simulink model "gm_parallel_8_prediction_and_cost_function"  (R2022a)
settings: Solver=FixedStepDiscrete  StartTime=0.0  StopTime=10.0  RelTol=1e-3
undefined symbols (not defined in the file or in its folder): f_c, L_d, L_q, L_x, L_y, p, psi_pm, R_ph
libraries: hdlmdlgenlib x42, hdlsllib x5
(part 2 of 7)

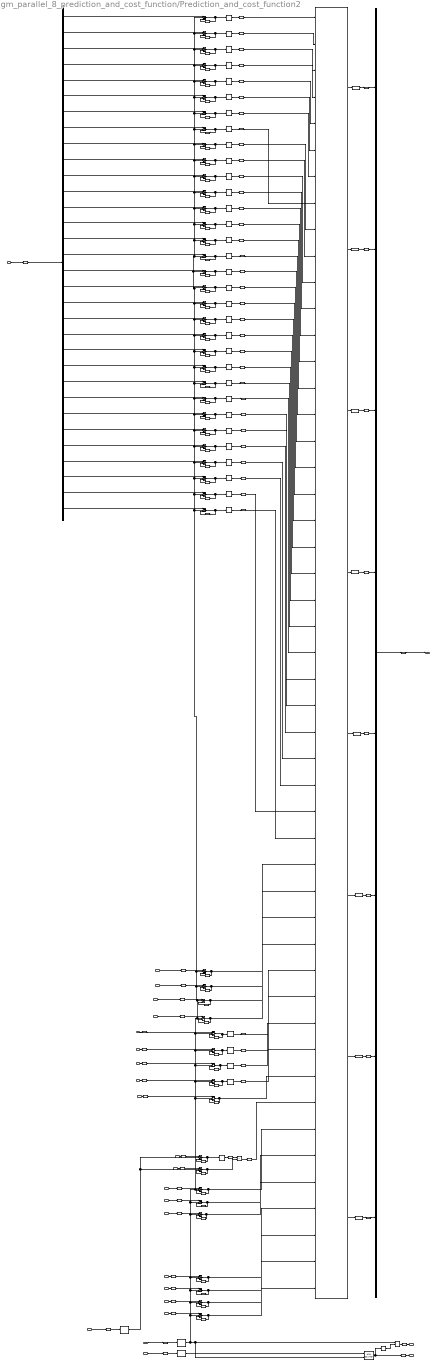
== system gm_parallel_8_prediction_and_cost_function/Prediction_and_cost_function2 ==
  Lq_AXI : Inport
  Ld_AXI : Inport  Port=2
  SampleTime_div_Ld_AXI : Inport  Port=3
  SampleTime_div_Lq_AXI : Inport  Port=4
  SampleTime_div_Lx_AXI : Inport  Port=5
  SampleTime_div_Ly_AXI : Inport  Port=6
  id_k_1 : Inport  Port=7
  iq_k_1 : Inport  Port=8
  ix_k_1 : Inport  Port=9
  iy_k_1 : Inport  Port=10
  Rs_AXI : Inport  Port=11
  omega_m_measured : Inport  Port=12
  pole_pairs_AXI : Inport  Port=13
  psiPM_AXI : Inport  Port=14
  id_ref_AXI : Inport  Port=15
  iq_ref_AXI : Inport  Port=16
  ix_ref_AXI : Inport  Port=17
  iy_ref_AXI : Inport  Port=18
  done_phase_voltages : Inport  Port=19
  done_vsd_and_park : Inport  Port=20
  current_valid_in : Inport  Port=21
  dqxy_phase_voltage_per_switching_state : Inport  Port=22
  Compare To Constant : hdlsllib/Logic and Bit Operations/Compare To Constant  relop=<=  const=8  OutDataTypeStr=boolean
      settings: SourceProductBaseCode=SL
  Data Type Conversion{4,7..10,18,39..45,53,55..77} (37 alike) : DataTypeConversion  OutDataTypeStr=single  RndMeth=Nearest  SaturateOnIntegerOverflow=off
  Data Type Conversion{46..52,54} (8 alike) : DataTypeConversion  OutDataTypeStr=fixdt(1,20,9)  SaturateOnIntegerOverflow=off  RndMeth=Floor
  Delay{1..4,8..37,42..45,51,57,59..60,68,104..135} (75 alike) : Delay  DelayLength=1
  Delay{5..7,38..41,46..50,52..56,58,61..67,69..89} (46 alike) : Delay  DelayLength=6
  Demux : Demux  Outputs=32
  Detect Rise Positive : hdlsllib/Logic and Bit Operations/Detect Rise Positive  vinit=0  OutDataTypeStr=boolean
      settings: SourceProductBaseCode=SL
  Detect Rise Positive1 : hdlsllib/Logic and Bit Operations/Detect Rise Positive  vinit=0  OutDataTypeStr=boolean
      settings: SourceProductBaseCode=SL
  Detect Rise Positive2 : hdlsllib/Logic and Bit Operations/Detect Rise Positive  vinit=0  OutDataTypeStr=boolean
      settings: SourceProductBaseCode=SL
  HDL Counter : hdlsllib/Sources/HDL Counter  CountType=Free running  CountInit=0  CountStep=1  CountMax=25  CountFromType=Initial value  CountFrom=0  CountResetPort=on  CountLoadPort=off  CountEnbPort=on  CountDirPort=off  CountHitOutputPort=off  CountDataType=Signed  CountWordLen=32  CountFracLen=0  CountSampTime=1
  Logical Operator : Logic  AllPortsSameDT=off  OutDataTypeStr=boolean
  Mux : Mux  Inputs=8
  Product : Product  Inputs=**
  Subsystem : Subsystem
  Switch_on{1..4,8..21,59..90} (50 alike) : Switch  Threshold=1  RndMeth=Simplest  SaturateOnIntegerOverflow=off  InputSameDT=off  OutDataTypeStr=Inherit: Same as first input
  done_Prediction_and_cost_function : Outport
  Index : Outport  Port=2
  J : Outport  Port=3
  wires:
  Delay89/1 -> Mux/8
  Delay88/1 -> Mux/7
  Delay87/1 -> Mux/6
  Delay86/1 -> Mux/5
  Delay85/1 -> Mux/4
  Delay84/1 -> Mux/3
  Delay83/1 -> Mux/2
  Delay82/1 -> Mux/1
  Delay81/1 -> Subsystem/1(d_phase_voltage_per_switching_state)
  Delay80/1 -> Subsystem/2(q_phase_voltage_per_switching_state)
  Delay79/1 -> Subsystem/3(x_phase_voltage_per_switching_state)
  Delay78/1 -> Subsystem/4(y_phase_voltage_per_switching_state)
  Delay77/1 -> Subsystem/5(d_phase_voltage_per_switching_state1)
  Delay76/1 -> Subsystem/6(q_phase_voltage_per_switching_state1)
  Delay75/1 -> Subsystem/7(x_phase_voltage_per_switching_state1)
  Delay74/1 -> Subsystem/8(y_phase_voltage_per_switching_state1)
  Delay73/1 -> Subsystem/9(d_phase_voltage_per_switching_state2)
  Delay72/1 -> Subsystem/10(q_phase_voltage_per_switching_state2)
  Delay71/1 -> Subsystem/11(x_phase_voltage_per_switching_state2)
  Delay70/1 -> Subsystem/12(y_phase_voltage_per_switching_state2)
  Delay69/1 -> Subsystem/13(d_phase_voltage_per_switching_state3)
  Delay67/1 -> Subsystem/14(q_phase_voltage_per_switching_state3)
  Delay66/1 -> Subsystem/15(x_phase_voltage_per_switching_state3)
  Delay65/1 -> Subsystem/16(y_phase_voltage_per_switching_state3)
  Delay64/1 -> Subsystem/17(d_phase_voltage_per_switching_state4)
  Delay63/1 -> Subsystem/18(q_phase_voltage_per_switching_state4)
  Delay62/1 -> Subsystem/19(x_phase_voltage_per_switching_state4)
  Delay61/1 -> Subsystem/20(y_phase_voltage_per_switching_state4)
  Delay58/1 -> Subsystem/21(d_phase_voltage_per_switching_state5)
  Delay56/1 -> Subsystem/22(q_phase_voltage_per_switching_state5)
  Delay55/1 -> Subsystem/23(x_phase_voltage_per_switching_state5)
  Delay54/1 -> Subsystem/24(y_phase_voltage_per_switching_state5)
  Delay53/1 -> Subsystem/25(d_phase_voltage_per_switching_state6)
  Delay52/1 -> Subsystem/26(q_phase_voltage_per_switching_state6)
  Delay50/1 -> Subsystem/27(x_phase_voltage_per_switching_state6)
  Delay49/1 -> Subsystem/28(y_phase_voltage_per_switching_state6)
  Delay48/1 -> Subsystem/29(d_phase_voltage_per_switching_state7)
  Delay47/1 -> Subsystem/30(q_phase_voltage_per_switching_state7)
  Delay46/1 -> Subsystem/31(x_phase_voltage_per_switching_state7)
  Delay41/1 -> Subsystem/32(y_phase_voltage_per_switching_state7)
  Data Type Conversion77/1 -> Delay81/1
  Data Type Conversion76/1 -> Delay80/1
  Data Type Conversion75/1 -> Delay79/1
  Data Type Conversion74/1 -> Delay78/1
  Data Type Conversion73/1 -> Delay77/1
  Data Type Conversion72/1 -> Delay76/1
  Data Type Conversion71/1 -> Delay75/1
  Data Type Conversion70/1 -> Delay74/1
  Data Type Conversion69/1 -> Delay73/1
  Data Type Conversion68/1 -> Delay72/1
  Data Type Conversion67/1 -> Delay71/1
  Data Type Conversion66/1 -> Delay70/1
  Data Type Conversion65/1 -> Delay69/1
  Data Type Conversion64/1 -> Delay67/1
  Data Type Conversion63/1 -> Delay66/1
  Data Type Conversion62/1 -> Delay65/1
  Data Type Conversion61/1 -> Delay64/1
  Data Type Conversion60/1 -> Delay63/1
  Data Type Conversion59/1 -> Delay62/1
  Data Type Conversion58/1 -> Delay61/1
  Data Type Conversion57/1 -> Delay58/1
  Data Type Conversion56/1 -> Delay56/1
  Data Type Conversion55/1 -> Delay55/1
  Data Type Conversion53/1 -> Delay54/1
  Data Type Conversion45/1 -> Delay53/1
  Data Type Conversion44/1 -> Delay52/1
  Data Type Conversion43/1 -> Delay50/1
  Data Type Conversion42/1 -> Delay49/1
  Data Type Conversion10/1 -> Delay48/1
  Data Type Conversion9/1 -> Delay47/1
  Data Type Conversion8/1 -> Delay46/1
  Data Type Conversion7/1 -> Delay41/1
  Delay40/1 -> Subsystem/37(id_k_16)
  Delay39/1 -> Subsystem/38(iq_k_16)
  Delay38/1 -> Subsystem/39(ix_k_16)
  Delay7/1 -> Subsystem/40(iy_k_16)
  Data Type Conversion41/1 -> Delay40/1
  Data Type Conversion40/1 -> Delay39/1
  Data Type Conversion39/1 -> Delay38/1
  Data Type Conversion18/1 -> Delay7/1
  Delay30/1 -> Switch_on13/1
  Delay6/1 -> Subsystem/42(omega_el15)
  Delay5/1 -> Product/1
  Data Type Conversion52/1 -> Delay89/1  "fc"
  Data Type Conversion51/1 -> Delay88/1  "fc"
  Data Type Conversion50/1 -> Delay87/1  "fc"
  Data Type Conversion49/1 -> Delay86/1  "fc"
  Data Type Conversion48/1 -> Delay85/1  "fc"
  Data Type Conversion47/1 -> Delay84/1  "fc"
  Data Type Conversion46/1 -> Delay83/1  "fc"
  Data Type Conversion54/1 -> Delay82/1  "fc"
  Subsystem/1(J) -> Data Type Conversion54/1  "fc"
  Subsystem/2(J1) -> Data Type Conversion46/1  "fc"
  Subsystem/3(J2) -> Data Type Conversion47/1  "fc"
  Subsystem/4(J3) -> Data Type Conversion48/1  "fc"
  Subsystem/5(J4) -> Data Type Conversion49/1  "fc"
  Subsystem/6(J5) -> Data Type Conversion50/1  "fc"
  Subsystem/7(J6) -> Data Type Conversion51/1  "fc"
  Subsystem/8(J7) -> Data Type Conversion52/1  "fc"
  Delay4/1 -> Switch_on4/3
  Switch_on4/1 -> Delay4/1, Product/2
  Detect Rise Positive2/1 -> Switch_on11/2, Switch_on4/2  "End_Cycle"
  Demux/1 -> Switch_on90/1
  Demux/2 -> Switch_on89/1
  Demux/3 -> Switch_on88/1
  Demux/4 -> Switch_on87/1
  Demux/5 -> Switch_on86/1
  Demux/6 -> Switch_on85/1
  Demux/7 -> Switch_on84/1
  Demux/8 -> Switch_on83/1
  Demux/9 -> Switch_on82/1
  Demux/10 -> Switch_on81/1
  Demux/11 -> Switch_on80/1
  Demux/12 -> Switch_on79/1
  Demux/13 -> Switch_on78/1
  Demux/14 -> Switch_on77/1
  Demux/15 -> Switch_on76/1
  Demux/16 -> Switch_on75/1
  Demux/17 -> Switch_on74/1
  Demux/18 -> Switch_on73/1
  Demux/19 -> Switch_on72/1
  Demux/20 -> Switch_on71/1
  Demux/21 -> Switch_on70/1
  Demux/22 -> Switch_on69/1
  Demux/23 -> Switch_on68/1
  Demux/24 -> Switch_on67/1
  Demux/25 -> Switch_on66/1
  Demux/26 -> Switch_on65/1
  Demux/27 -> Switch_on64/1
  Demux/28 -> Switch_on63/1
  Demux/29 -> Switch_on62/1
  Demux/30 -> Switch_on61/1
  Demux/31 -> Switch_on60/1
  Demux/32 -> Switch_on59/1
  Data Type Conversion4/1 -> Delay5/1
  Delay27/1 -> Switch_on17/1
  Delay28/1 -> Switch_on16/1
  Delay29/1 -> Switch_on15/1
  Delay32/1 -> Demux/1
  Delay22/1 -> done_Prediction_and_cost_function/1
  dqxy_phase_voltage_per_switching_state/1 -> Delay32/1
  Detect Rise Positive/1 -> Switch_on2/2, Switch_on3/2, Switch_on10/2, Switch_on13/2, Switch_on15/2, Switch_on16/2, Switch_on17/2, Switch_on18/2, Switch_on19/2, Switch_on21/2, Switch_on59/2, Switch_on60/2, Switch_on61/2, Switch_on62/2, Switch_on63/2, Switch_on64/2, Switch_on65/2, Switch_on66/2, Switch_on67/2, Switch_on68/2, Switch_on69/2, Switch_on70/2, Switch_on71/2, Switch_on72/2, Switch_on73/2, Switch_on74/2, Switch_on75/2, Switch_on76/2, Switch_on77/2, Switch_on78/2, Switch_on79/2, Switch_on80/2, Switch_on81/2, Switch_on82/2, Switch_on83/2, Switch_on84/2, Switch_on85/2, Switch_on86/2, Switch_on87/2, Switch_on88/2, Switch_on89/2, Switch_on90/2, Switch_on20/2, Switch_on12/2, Switch_on9/2, Switch_on8/2, Switch_on1/2, Switch_on14/2, HDL Counter/2, Logical Operator/1  "End_Cycle"
  Switch_on88/1 -> Delay133/1, Data Type Conversion75/1
  Delay133/1 -> Switch_on88/3
  Switch_on87/1 -> Delay132/1, Data Type Conversion74/1
  Delay132/1 -> Switch_on87/3
  Switch_on90/1 -> Delay135/1, Data Type Conversion77/1
  Delay135/1 -> Switch_on90/3
  Delay134/1 -> Switch_on89/3
  Switch_on89/1 -> Delay134/1, Data Type Conversion76/1
  Switch_on84/1 -> Delay129/1, Data Type Conversion71/1
  Delay129/1 -> Switch_on84/3
  Switch_on83/1 -> Delay128/1, Data Type Conversion70/1
  Delay128/1 -> Switch_on83/3
  Switch_on86/1 -> Delay131/1, Data Type Conversion73/1
  Delay131/1 -> Switch_on86/3
  Delay130/1 -> Switch_on85/3
  Switch_on85/1 -> Delay130/1, Data Type Conversion72/1
  Switch_on80/1 -> Delay125/1, Data Type Conversion67/1
  Delay125/1 -> Switch_on80/3
  Switch_on79/1 -> Delay124/1, Data Type Conversion66/1
  Delay124/1 -> Switch_on79/3
  Switch_on82/1 -> Delay127/1, Data Type Conversion69/1
  Delay127/1 -> Switch_on82/3
  Delay126/1 -> Switch_on81/3
  Switch_on81/1 -> Delay126/1, Data Type Conversion68/1
  Switch_on76/1 -> Delay121/1, Data Type Conversion63/1
  Delay121/1 -> Switch_on76/3
  Switch_on75/1 -> Delay120/1, Data Type Conversion62/1
  Delay120/1 -> Switch_on75/3
  Switch_on78/1 -> Delay123/1, Data Type Conversion65/1
  Delay123/1 -> Switch_on78/3
  Delay122/1 -> Switch_on77/3
  Switch_on77/1 -> Delay122/1, Data Type Conversion64/1
  Switch_on72/1 -> Delay117/1, Data Type Conversion59/1
  Delay117/1 -> Switch_on72/3
  Switch_on71/1 -> Delay116/1, Data Type Conversion58/1
  Delay116/1 -> Switch_on71/3
  Switch_on74/1 -> Delay119/1, Data Type Conversion61/1
  Delay119/1 -> Switch_on74/3
  Delay118/1 -> Switch_on73/3
  Switch_on73/1 -> Delay118/1, Data Type Conversion60/1
  Switch_on68/1 -> Delay113/1, Data Type Conversion55/1
  Delay113/1 -> Switch_on68/3
  Switch_on67/1 -> Delay112/1, Data Type Conversion53/1
  Delay112/1 -> Switch_on67/3
  Switch_on70/1 -> Delay115/1, Data Type Conversion57/1
  Delay115/1 -> Switch_on70/3
  Delay114/1 -> Switch_on69/3
  Switch_on69/1 -> Delay114/1, Data Type Conversion56/1
  Switch_on64/1 -> Delay109/1, Data Type Conversion43/1
  Delay109/1 -> Switch_on64/3
  Switch_on63/1 -> Delay108/1, Data Type Conversion42/1
  Delay108/1 -> Switch_on63/3
  Switch_on66/1 -> Delay111/1, Data Type Conversion45/1
  Delay111/1 -> Switch_on66/3
  Delay110/1 -> Switch_on65/3
  Switch_on65/1 -> Delay110/1, Data Type Conversion44/1
  Switch_on60/1 -> Delay105/1, Data Type Conversion8/1
  Delay105/1 -> Switch_on60/3
  Switch_on59/1 -> Delay104/1, Data Type Conversion7/1
  Delay104/1 -> Switch_on59/3
  Switch_on62/1 -> Delay107/1, Data Type Conversion10/1
  Delay107/1 -> Switch_on62/3
  Delay106/1 -> Switch_on61/3
  Switch_on61/1 -> Delay106/1, Data Type Conversion9/1
  Delay68/1 -> J/1
  Mux/1 -> Delay68/1
  Delay60/1 -> Detect Rise Positive2/1
  current_valid_in/1 -> Delay60/1
  Delay59/1 -> Index/1
  Logical Operator/1 -> Delay22/1
  Compare To Constant/1 -> Logical Operator/2
  HDL Counter/1 -> Delay59/1, Compare To Constant/1
  Detect Rise Positive1/1 -> HDL Counter/1  "End_Cycle"
  Delay57/1 -> Detect Rise Positive1/1
  done_vsd_and_park/1 -> Delay57/1
  SampleTime_div_Ly_AXI/1 -> Delay26/1
  SampleTime_div_Lx_AXI/1 -> Delay25/1
  SampleTime_div_Lq_AXI/1 -> Delay24/1
  SampleTime_div_Ld_AXI/1 -> Delay23/1
  Delay51/1 -> Switch_on11/1
  Delay8/1 -> Switch_on8/3
  Switch_on8/1 -> Subsystem/45(psiPM15), Delay8/1
  Delay44/1 -> Switch_on1/1
  id_ref_AXI/1 -> Delay42/1
  Delay14/1 -> Switch_on15/3
  Delay26/1 -> Switch_on18/1
  Switch_on9/1 -> Subsystem/44(Ld15), Delay9/1
  ix_ref_AXI/1 -> Delay44/1
  id_k_1/1 -> Delay27/1
  Switch_on1/1 -> Subsystem/48(ix_ref15), Delay1/1
  iy_ref_AXI/1 -> Delay45/1
  Delay34/1 -> Switch_on10/1
  Switch_on2/1 -> Subsystem/47(iq_ref15), Delay2/1
  Switch_on21/1 -> Subsystem/33(SampleTime_div_Ld15), Delay20/1
  Switch_on3/1 -> Subsystem/46(id_ref15), Delay3/1
  Delay21/1 -> Detect Rise Positive/1
  Delay12/1 -> Switch_on12/3
  Switch_on14/1 -> Subsystem/49(iy_ref15), Delay33/1
  psiPM_AXI/1 -> Delay37/1
  Delay25/1 -> Switch_on19/1
  Ld_AXI/1 -> Delay36/1
  Delay33/1 -> Switch_on14/3
  Switch_on11/1 -> Delay11/1, Data Type Conversion4/1
  iq_ref_AXI/1 -> Delay43/1
  Switch_on16/1 -> Data Type Conversion40/1, Delay15/1
  Delay15/1 -> Switch_on16/3
  iq_k_1/1 -> Delay28/1
  Switch_on17/1 -> Data Type Conversion41/1, Delay16/1
  Delay16/1 -> Switch_on17/3
  Delay2/1 -> Switch_on2/3
  Delay45/1 -> Switch_on14/1
  ix_k_1/1 -> Delay29/1
  Switch_on13/1 -> Data Type Conversion18/1, Delay13/1
  Switch_on20/1 -> Subsystem/34(SampleTime_div_Lq15), Delay19/1
  Switch_on19/1 -> Subsystem/35(SampleTime_div_Lx15), Delay18/1
  Lq_AXI/1 -> Delay34/1
  Delay18/1 -> Switch_on19/3
  Switch_on15/1 -> Data Type Conversion39/1, Delay14/1
  Delay13/1 -> Switch_on13/3
  Delay19/1 -> Switch_on20/3
  Switch_on18/1 -> Subsystem/36(SampleTime_div_Ly15), Delay17/1
  omega_m_measured/1 -> Delay51/1
  pole_pairs_AXI/1 -> Delay35/1
  Delay35/1 -> Switch_on4/1
  Delay20/1 -> Switch_on21/3
  iy_k_1/1 -> Delay30/1
  Delay9/1 -> Switch_on9/3
  done_phase_voltages/1 -> Delay21/1
  Product/1 -> Delay6/1  "omega_el"
  Delay42/1 -> Switch_on3/1
  Delay1/1 -> Switch_on1/3
  Delay37/1 -> Switch_on8/1
  Delay36/1 -> Switch_on9/1
  Delay24/1 -> Switch_on20/1
  Delay11/1 -> Switch_on11/3
  Switch_on10/1 -> Subsystem/43(Lq15), Delay10/1
  Delay17/1 -> Switch_on18/3
  Delay43/1 -> Switch_on2/1
  Delay10/1 -> Switch_on10/3
  Delay3/1 -> Switch_on3/3
  Delay23/1 -> Switch_on21/1
  Delay31/1 -> Switch_on12/1
  Rs_AXI/1 -> Delay31/1
  Switch_on12/1 -> Delay12/1, Subsystem/41(Rs15)

== system gm_parallel_8_prediction_and_cost_function/Prediction_and_cost_function1/Compare To Constant ==
  u : Inport  OutDataTypeStr=fixdt(1,32,0,'DataTypeOverride', 'Off')  SampleTime=1e-08
  Compare : RelationalOperator  Operator=<=  OutDataTypeStr=boolean
  Constant : Constant  DisableCoverage=on  Value=const  OutDataTypeStr=Inherit: Inherit via back propagation  SampleTime=-1
  y : Outport  SampleTime=1e-08
  wires:
  Compare/1 -> y/1
  Constant/1 -> Compare/2
  u/1 -> Compare/1

== system gm_parallel_8_prediction_and_cost_function/Prediction_and_cost_function1/Data Type Conversion10 ==
  In1 : Inport
  Data Type Conversion10 : DataTypeConversion  OutDataTypeStr=single  RndMeth=Nearest  SampleTime=1e-08  SaturateOnIntegerOverflow=off
  Data Type Conversion10_pd1 : Delay  DelayLength=6
  Out1 : Outport
  wires:
  In1/1 -> Data Type Conversion10/1
  Data Type Conversion10/1 -> Data Type Conversion10_pd1/1
  Data Type Conversion10_pd1/1 -> Out1/1

== system gm_parallel_8_prediction_and_cost_function/Prediction_and_cost_function1/Data Type Conversion18 ==
  In1 : Inport
  Data Type Conversion18 : DataTypeConversion  OutDataTypeStr=single  RndMeth=Nearest  SampleTime=1e-08  SaturateOnIntegerOverflow=off
  Data Type Conversion18_pd1 : Delay  DelayLength=6
  Out1 : Outport
  wires:
  In1/1 -> Data Type Conversion18/1
  Data Type Conversion18/1 -> Data Type Conversion18_pd1/1
  Data Type Conversion18_pd1/1 -> Out1/1

== system gm_parallel_8_prediction_and_cost_function/Prediction_and_cost_function1/Data Type Conversion39 ==
  In1 : Inport
  Data Type Conversion39 : DataTypeConversion  OutDataTypeStr=single  RndMeth=Nearest  SampleTime=1e-08  SaturateOnIntegerOverflow=off
  Data Type Conversion39_pd1 : Delay  DelayLength=6
  Out1 : Outport
  wires:
  In1/1 -> Data Type Conversion39/1
  Data Type Conversion39/1 -> Data Type Conversion39_pd1/1
  Data Type Conversion39_pd1/1 -> Out1/1

== system gm_parallel_8_prediction_and_cost_function/Prediction_and_cost_function1/Data Type Conversion4 ==
  In1 : Inport
  Data Type Conversion4 : DataTypeConversion  OutDataTypeStr=single  RndMeth=Nearest  SampleTime=1e-08  SaturateOnIntegerOverflow=off
  Data Type Conversion4_pd1 : Delay  DelayLength=6
  Out1 : Outport
  wires:
  In1/1 -> Data Type Conversion4/1
  Data Type Conversion4/1 -> Data Type Conversion4_pd1/1
  Data Type Conversion4_pd1/1 -> Out1/1

== system gm_parallel_8_prediction_and_cost_function/Prediction_and_cost_function1/Data Type Conversion40 ==
  In1 : Inport
  Data Type Conversion40 : DataTypeConversion  OutDataTypeStr=single  RndMeth=Nearest  SampleTime=1e-08  SaturateOnIntegerOverflow=off
  Data Type Conversion40_pd1 : Delay  DelayLength=6
  Out1 : Outport
  wires:
  In1/1 -> Data Type Conversion40/1
  Data Type Conversion40/1 -> Data Type Conversion40_pd1/1
  Data Type Conversion40_pd1/1 -> Out1/1

== system gm_parallel_8_prediction_and_cost_function/Prediction_and_cost_function1/Data Type Conversion41 ==
  In1 : Inport
  Data Type Conversion41 : DataTypeConversion  OutDataTypeStr=single  RndMeth=Nearest  SampleTime=1e-08  SaturateOnIntegerOverflow=off
  Data Type Conversion41_pd1 : Delay  DelayLength=6
  Out1 : Outport
  wires:
  In1/1 -> Data Type Conversion41/1
  Data Type Conversion41/1 -> Data Type Conversion41_pd1/1
  Data Type Conversion41_pd1/1 -> Out1/1

== system gm_parallel_8_prediction_and_cost_function/Prediction_and_cost_function1/Data Type Conversion42 ==
  In1 : Inport
  Data Type Conversion42 : DataTypeConversion  OutDataTypeStr=single  RndMeth=Nearest  SampleTime=1e-08  SaturateOnIntegerOverflow=off
  Data Type Conversion42_pd1 : Delay  DelayLength=6
  Out1 : Outport
  wires:
  In1/1 -> Data Type Conversion42/1
  Data Type Conversion42/1 -> Data Type Conversion42_pd1/1
  Data Type Conversion42_pd1/1 -> Out1/1

== system gm_parallel_8_prediction_and_cost_function/Prediction_and_cost_function1/Data Type Conversion43 ==
  In1 : Inport
  Data Type Conversion43 : DataTypeConversion  OutDataTypeStr=single  RndMeth=Nearest  SampleTime=1e-08  SaturateOnIntegerOverflow=off
  Data Type Conversion43_pd1 : Delay  DelayLength=6
  Out1 : Outport
  wires:
  In1/1 -> Data Type Conversion43/1
  Data Type Conversion43/1 -> Data Type Conversion43_pd1/1
  Data Type Conversion43_pd1/1 -> Out1/1

== system gm_parallel_8_prediction_and_cost_function/Prediction_and_cost_function1/Data Type Conversion44 ==
  In1 : Inport
  Data Type Conversion44 : DataTypeConversion  OutDataTypeStr=single  RndMeth=Nearest  SampleTime=1e-08  SaturateOnIntegerOverflow=off
  Data Type Conversion44_pd1 : Delay  DelayLength=6
  Out1 : Outport
  wires:
  In1/1 -> Data Type Conversion44/1
  Data Type Conversion44/1 -> Data Type Conversion44_pd1/1
  Data Type Conversion44_pd1/1 -> Out1/1

== system gm_parallel_8_prediction_and_cost_function/Prediction_and_cost_function1/Data Type Conversion45 ==
  In1 : Inport
  Data Type Conversion45 : DataTypeConversion  OutDataTypeStr=single  RndMeth=Nearest  SampleTime=1e-08  SaturateOnIntegerOverflow=off
  Data Type Conversion45_pd1 : Delay  DelayLength=6
  Out1 : Outport
  wires:
  In1/1 -> Data Type Conversion45/1
  Data Type Conversion45/1 -> Data Type Conversion45_pd1/1
  Data Type Conversion45_pd1/1 -> Out1/1

== system gm_parallel_8_prediction_and_cost_function/Prediction_and_cost_function1/Data Type Conversion46 ==
  In1 : Inport
  Data Type Conversion46 : DataTypeConversion  OutDataTypeStr=fixdt(1, 20, 9)  SampleTime=1e-08  SaturateOnIntegerOverflow=off  RndMeth=Floor
  Data Type Conversion46_pd1 : Delay  DelayLength=6
  Out1 : Outport
  wires:
  In1/1 -> Data Type Conversion46/1
  Data Type Conversion46/1 -> Data Type Conversion46_pd1/1
  Data Type Conversion46_pd1/1 -> Out1/1

== system gm_parallel_8_prediction_and_cost_function/Prediction_and_cost_function1/Data Type Conversion47 ==
  In1 : Inport
  Data Type Conversion47 : DataTypeConversion  OutDataTypeStr=fixdt(1, 20, 9)  SampleTime=1e-08  SaturateOnIntegerOverflow=off  RndMeth=Floor
  Data Type Conversion47_pd1 : Delay  DelayLength=6
  Out1 : Outport
  wires:
  In1/1 -> Data Type Conversion47/1
  Data Type Conversion47/1 -> Data Type Conversion47_pd1/1
  Data Type Conversion47_pd1/1 -> Out1/1

== system gm_parallel_8_prediction_and_cost_function/Prediction_and_cost_function1/Data Type Conversion48 ==
  In1 : Inport
  Data Type Conversion48 : DataTypeConversion  OutDataTypeStr=fixdt(1, 20, 9)  SampleTime=1e-08  SaturateOnIntegerOverflow=off  RndMeth=Floor
  Data Type Conversion48_pd1 : Delay  DelayLength=6
  Out1 : Outport
  wires:
  In1/1 -> Data Type Conversion48/1
  Data Type Conversion48/1 -> Data Type Conversion48_pd1/1
  Data Type Conversion48_pd1/1 -> Out1/1

== system gm_parallel_8_prediction_and_cost_function/Prediction_and_cost_function1/Data Type Conversion49 ==
  In1 : Inport
  Data Type Conversion49 : DataTypeConversion  OutDataTypeStr=fixdt(1, 20, 9)  SampleTime=1e-08  SaturateOnIntegerOverflow=off  RndMeth=Floor
  Data Type Conversion49_pd1 : Delay  DelayLength=6
  Out1 : Outport
  wires:
  In1/1 -> Data Type Conversion49/1
  Data Type Conversion49/1 -> Data Type Conversion49_pd1/1
  Data Type Conversion49_pd1/1 -> Out1/1

== system gm_parallel_8_prediction_and_cost_function/Prediction_and_cost_function1/Data Type Conversion50 ==
  In1 : Inport
  Data Type Conversion50 : DataTypeConversion  OutDataTypeStr=fixdt(1, 20, 9)  SampleTime=1e-08  SaturateOnIntegerOverflow=off  RndMeth=Floor
  Data Type Conversion50_pd1 : Delay  DelayLength=6
  Out1 : Outport
  wires:
  In1/1 -> Data Type Conversion50/1
  Data Type Conversion50/1 -> Data Type Conversion50_pd1/1
  Data Type Conversion50_pd1/1 -> Out1/1

== system gm_parallel_8_prediction_and_cost_function/Prediction_and_cost_function1/Data Type Conversion51 ==
  In1 : Inport
  Data Type Conversion51 : DataTypeConversion  OutDataTypeStr=fixdt(1, 20, 9)  SampleTime=1e-08  SaturateOnIntegerOverflow=off  RndMeth=Floor
  Data Type Conversion51_pd1 : Delay  DelayLength=6
  Out1 : Outport
  wires:
  In1/1 -> Data Type Conversion51/1
  Data Type Conversion51/1 -> Data Type Conversion51_pd1/1
  Data Type Conversion51_pd1/1 -> Out1/1

== system gm_parallel_8_prediction_and_cost_function/Prediction_and_cost_function1/Data Type Conversion52 ==
  In1 : Inport
  Data Type Conversion52 : DataTypeConversion  OutDataTypeStr=fixdt(1, 20, 9)  SampleTime=1e-08  SaturateOnIntegerOverflow=off  RndMeth=Floor
  Data Type Conversion52_pd1 : Delay  DelayLength=6
  Out1 : Outport
  wires:
  In1/1 -> Data Type Conversion52/1
  Data Type Conversion52/1 -> Data Type Conversion52_pd1/1
  Data Type Conversion52_pd1/1 -> Out1/1

== system gm_parallel_8_prediction_and_cost_function/Prediction_and_cost_function1/Data Type Conversion53 ==
  In1 : Inport
  Data Type Conversion53 : DataTypeConversion  OutDataTypeStr=single  RndMeth=Nearest  SampleTime=1e-08  SaturateOnIntegerOverflow=off
  Data Type Conversion53_pd1 : Delay  DelayLength=6
  Out1 : Outport
  wires:
  In1/1 -> Data Type Conversion53/1
  Data Type Conversion53/1 -> Data Type Conversion53_pd1/1
  Data Type Conversion53_pd1/1 -> Out1/1

== system gm_parallel_8_prediction_and_cost_function/Prediction_and_cost_function1/Data Type Conversion54 ==
  In1 : Inport
  Data Type Conversion54 : DataTypeConversion  OutDataTypeStr=fixdt(1, 20, 9)  SampleTime=1e-08  SaturateOnIntegerOverflow=off  RndMeth=Floor
  Data Type Conversion54_pd1 : Delay  DelayLength=6
  Out1 : Outport
  wires:
  In1/1 -> Data Type Conversion54/1
  Data Type Conversion54/1 -> Data Type Conversion54_pd1/1
  Data Type Conversion54_pd1/1 -> Out1/1

== system gm_parallel_8_prediction_and_cost_function/Prediction_and_cost_function1/Data Type Conversion55 ==
  In1 : Inport
  Data Type Conversion55 : DataTypeConversion  OutDataTypeStr=single  RndMeth=Nearest  SampleTime=1e-08  SaturateOnIntegerOverflow=off
  Data Type Conversion55_pd1 : Delay  DelayLength=6
  Out1 : Outport
  wires:
  In1/1 -> Data Type Conversion55/1
  Data Type Conversion55/1 -> Data Type Conversion55_pd1/1
  Data Type Conversion55_pd1/1 -> Out1/1

== system gm_parallel_8_prediction_and_cost_function/Prediction_and_cost_function1/Data Type Conversion56 ==
  In1 : Inport
  Data Type Conversion56 : DataTypeConversion  OutDataTypeStr=single  RndMeth=Nearest  SampleTime=1e-08  SaturateOnIntegerOverflow=off
  Data Type Conversion56_pd1 : Delay  DelayLength=6
  Out1 : Outport
  wires:
  In1/1 -> Data Type Conversion56/1
  Data Type Conversion56/1 -> Data Type Conversion56_pd1/1
  Data Type Conversion56_pd1/1 -> Out1/1

== system gm_parallel_8_prediction_and_cost_function/Prediction_and_cost_function1/Data Type Conversion57 ==
  In1 : Inport
  Data Type Conversion57 : DataTypeConversion  OutDataTypeStr=single  RndMeth=Nearest  SampleTime=1e-08  SaturateOnIntegerOverflow=off
  Data Type Conversion57_pd1 : Delay  DelayLength=6
  Out1 : Outport
  wires:
  In1/1 -> Data Type Conversion57/1
  Data Type Conversion57/1 -> Data Type Conversion57_pd1/1
  Data Type Conversion57_pd1/1 -> Out1/1

== system gm_parallel_8_prediction_and_cost_function/Prediction_and_cost_function1/Data Type Conversion58 ==
  In1 : Inport
  Data Type Conversion58 : DataTypeConversion  OutDataTypeStr=single  RndMeth=Nearest  SampleTime=1e-08  SaturateOnIntegerOverflow=off
  Data Type Conversion58_pd1 : Delay  DelayLength=6
  Out1 : Outport
  wires:
  In1/1 -> Data Type Conversion58/1
  Data Type Conversion58/1 -> Data Type Conversion58_pd1/1
  Data Type Conversion58_pd1/1 -> Out1/1

== system gm_parallel_8_prediction_and_cost_function/Prediction_and_cost_function1/Data Type Conversion59 ==
  In1 : Inport
  Data Type Conversion59 : DataTypeConversion  OutDataTypeStr=single  RndMeth=Nearest  SampleTime=1e-08  SaturateOnIntegerOverflow=off
  Data Type Conversion59_pd1 : Delay  DelayLength=6
  Out1 : Outport
  wires:
  In1/1 -> Data Type Conversion59/1
  Data Type Conversion59/1 -> Data Type Conversion59_pd1/1
  Data Type Conversion59_pd1/1 -> Out1/1

== system gm_parallel_8_prediction_and_cost_function/Prediction_and_cost_function1/Data Type Conversion60 ==
  In1 : Inport
  Data Type Conversion60 : DataTypeConversion  OutDataTypeStr=single  RndMeth=Nearest  SampleTime=1e-08  SaturateOnIntegerOverflow=off
  Data Type Conversion60_pd1 : Delay  DelayLength=6
  Out1 : Outport
  wires:
  In1/1 -> Data Type Conversion60/1
  Data Type Conversion60/1 -> Data Type Conversion60_pd1/1
  Data Type Conversion60_pd1/1 -> Out1/1

== system gm_parallel_8_prediction_and_cost_function/Prediction_and_cost_function1/Data Type Conversion61 ==
  In1 : Inport
  Data Type Conversion61 : DataTypeConversion  OutDataTypeStr=single  RndMeth=Nearest  SampleTime=1e-08  SaturateOnIntegerOverflow=off
  Data Type Conversion61_pd1 : Delay  DelayLength=6
  Out1 : Outport
  wires:
  In1/1 -> Data Type Conversion61/1
  Data Type Conversion61/1 -> Data Type Conversion61_pd1/1
  Data Type Conversion61_pd1/1 -> Out1/1

== system gm_parallel_8_prediction_and_cost_function/Prediction_and_cost_function1/Data Type Conversion62 ==
  In1 : Inport
  Data Type Conversion62 : DataTypeConversion  OutDataTypeStr=single  RndMeth=Nearest  SampleTime=1e-08  SaturateOnIntegerOverflow=off
  Data Type Conversion62_pd1 : Delay  DelayLength=6
  Out1 : Outport
  wires:
  In1/1 -> Data Type Conversion62/1
  Data Type Conversion62/1 -> Data Type Conversion62_pd1/1
  Data Type Conversion62_pd1/1 -> Out1/1

== system gm_parallel_8_prediction_and_cost_function/Prediction_and_cost_function1/Data Type Conversion63 ==
  In1 : Inport
  Data Type Conversion63 : DataTypeConversion  OutDataTypeStr=single  RndMeth=Nearest  SampleTime=1e-08  SaturateOnIntegerOverflow=off
  Data Type Conversion63_pd1 : Delay  DelayLength=6
  Out1 : Outport
  wires:
  In1/1 -> Data Type Conversion63/1
  Data Type Conversion63/1 -> Data Type Conversion63_pd1/1
  Data Type Conversion63_pd1/1 -> Out1/1

== system gm_parallel_8_prediction_and_cost_function/Prediction_and_cost_function1/Data Type Conversion64 ==
  In1 : Inport
  Data Type Conversion64 : DataTypeConversion  OutDataTypeStr=single  RndMeth=Nearest  SampleTime=1e-08  SaturateOnIntegerOverflow=off
  Data Type Conversion64_pd1 : Delay  DelayLength=6
  Out1 : Outport
  wires:
  In1/1 -> Data Type Conversion64/1
  Data Type Conversion64/1 -> Data Type Conversion64_pd1/1
  Data Type Conversion64_pd1/1 -> Out1/1

== system gm_parallel_8_prediction_and_cost_function/Prediction_and_cost_function1/Data Type Conversion65 ==
  In1 : Inport
  Data Type Conversion65 : DataTypeConversion  OutDataTypeStr=single  RndMeth=Nearest  SampleTime=1e-08  SaturateOnIntegerOverflow=off
  Data Type Conversion65_pd1 : Delay  DelayLength=6
  Out1 : Outport
  wires:
  In1/1 -> Data Type Conversion65/1
  Data Type Conversion65/1 -> Data Type Conversion65_pd1/1
  Data Type Conversion65_pd1/1 -> Out1/1

== system gm_parallel_8_prediction_and_cost_function/Prediction_and_cost_function1/Data Type Conversion66 ==
  In1 : Inport
  Data Type Conversion66 : DataTypeConversion  OutDataTypeStr=single  RndMeth=Nearest  SampleTime=1e-08  SaturateOnIntegerOverflow=off
  Data Type Conversion66_pd1 : Delay  DelayLength=6
  Out1 : Outport
  wires:
  In1/1 -> Data Type Conversion66/1
  Data Type Conversion66/1 -> Data Type Conversion66_pd1/1
  Data Type Conversion66_pd1/1 -> Out1/1

== system gm_parallel_8_prediction_and_cost_function/Prediction_and_cost_function1/Data Type Conversion67 ==
  In1 : Inport
  Data Type Conversion67 : DataTypeConversion  OutDataTypeStr=single  RndMeth=Nearest  SampleTime=1e-08  SaturateOnIntegerOverflow=off
  Data Type Conversion67_pd1 : Delay  DelayLength=6
  Out1 : Outport
  wires:
  In1/1 -> Data Type Conversion67/1
  Data Type Conversion67/1 -> Data Type Conversion67_pd1/1
  Data Type Conversion67_pd1/1 -> Out1/1

== system gm_parallel_8_prediction_and_cost_function/Prediction_and_cost_function1/Data Type Conversion68 ==
  In1 : Inport
  Data Type Conversion68 : DataTypeConversion  OutDataTypeStr=single  RndMeth=Nearest  SampleTime=1e-08  SaturateOnIntegerOverflow=off
  Data Type Conversion68_pd1 : Delay  DelayLength=6
  Out1 : Outport
  wires:
  In1/1 -> Data Type Conversion68/1
  Data Type Conversion68/1 -> Data Type Conversion68_pd1/1
  Data Type Conversion68_pd1/1 -> Out1/1

== system gm_parallel_8_prediction_and_cost_function/Prediction_and_cost_function1/Data Type Conversion69 ==
  In1 : Inport
  Data Type Conversion69 : DataTypeConversion  OutDataTypeStr=single  RndMeth=Nearest  SampleTime=1e-08  SaturateOnIntegerOverflow=off
  Data Type Conversion69_pd1 : Delay  DelayLength=6
  Out1 : Outport
  wires:
  In1/1 -> Data Type Conversion69/1
  Data Type Conversion69/1 -> Data Type Conversion69_pd1/1
  Data Type Conversion69_pd1/1 -> Out1/1

== system gm_parallel_8_prediction_and_cost_function/Prediction_and_cost_function1/Data Type Conversion7 ==
  In1 : Inport
  Data Type Conversion7 : DataTypeConversion  OutDataTypeStr=single  RndMeth=Nearest  SampleTime=1e-08  SaturateOnIntegerOverflow=off
  Data Type Conversion7_pd1 : Delay  DelayLength=6
  Out1 : Outport
  wires:
  In1/1 -> Data Type Conversion7/1
  Data Type Conversion7/1 -> Data Type Conversion7_pd1/1
  Data Type Conversion7_pd1/1 -> Out1/1

== system gm_parallel_8_prediction_and_cost_function/Prediction_and_cost_function1/Data Type Conversion70 ==
  In1 : Inport
  Data Type Conversion70 : DataTypeConversion  OutDataTypeStr=single  RndMeth=Nearest  SampleTime=1e-08  SaturateOnIntegerOverflow=off
  Data Type Conversion70_pd1 : Delay  DelayLength=6
  Out1 : Outport
  wires:
  In1/1 -> Data Type Conversion70/1
  Data Type Conversion70/1 -> Data Type Conversion70_pd1/1
  Data Type Conversion70_pd1/1 -> Out1/1

== system gm_parallel_8_prediction_and_cost_function/Prediction_and_cost_function1/Data Type Conversion71 ==
  In1 : Inport
  Data Type Conversion71 : DataTypeConversion  OutDataTypeStr=single  RndMeth=Nearest  SampleTime=1e-08  SaturateOnIntegerOverflow=off
  Data Type Conversion71_pd1 : Delay  DelayLength=6
  Out1 : Outport
  wires:
  In1/1 -> Data Type Conversion71/1
  Data Type Conversion71/1 -> Data Type Conversion71_pd1/1
  Data Type Conversion71_pd1/1 -> Out1/1

== system gm_parallel_8_prediction_and_cost_function/Prediction_and_cost_function1/Data Type Conversion72 ==
  In1 : Inport
  Data Type Conversion72 : DataTypeConversion  OutDataTypeStr=single  RndMeth=Nearest  SampleTime=1e-08  SaturateOnIntegerOverflow=off
  Data Type Conversion72_pd1 : Delay  DelayLength=6
  Out1 : Outport
  wires:
  In1/1 -> Data Type Conversion72/1
  Data Type Conversion72/1 -> Data Type Conversion72_pd1/1
  Data Type Conversion72_pd1/1 -> Out1/1

== system gm_parallel_8_prediction_and_cost_function/Prediction_and_cost_function1/Data Type Conversion73 ==
  In1 : Inport
  Data Type Conversion73 : DataTypeConversion  OutDataTypeStr=single  RndMeth=Nearest  SampleTime=1e-08  SaturateOnIntegerOverflow=off
  Data Type Conversion73_pd1 : Delay  DelayLength=6
  Out1 : Outport
  wires:
  In1/1 -> Data Type Conversion73/1
  Data Type Conversion73/1 -> Data Type Conversion73_pd1/1
  Data Type Conversion73_pd1/1 -> Out1/1

== system gm_parallel_8_prediction_and_cost_function/Prediction_and_cost_function1/Data Type Conversion74 ==
  In1 : Inport
  Data Type Conversion74 : DataTypeConversion  OutDataTypeStr=single  RndMeth=Nearest  SampleTime=1e-08  SaturateOnIntegerOverflow=off
  Data Type Conversion74_pd1 : Delay  DelayLength=6
  Out1 : Outport
  wires:
  In1/1 -> Data Type Conversion74/1
  Data Type Conversion74/1 -> Data Type Conversion74_pd1/1
  Data Type Conversion74_pd1/1 -> Out1/1

== system gm_parallel_8_prediction_and_cost_function/Prediction_and_cost_function1/Data Type Conversion75 ==
  In1 : Inport
  Data Type Conversion75 : DataTypeConversion  OutDataTypeStr=single  RndMeth=Nearest  SampleTime=1e-08  SaturateOnIntegerOverflow=off
  Data Type Conversion75_pd1 : Delay  DelayLength=6
  Out1 : Outport
  wires:
  In1/1 -> Data Type Conversion75/1
  Data Type Conversion75/1 -> Data Type Conversion75_pd1/1
  Data Type Conversion75_pd1/1 -> Out1/1

== system gm_parallel_8_prediction_and_cost_function/Prediction_and_cost_function1/Data Type Conversion76 ==
  In1 : Inport
  Data Type Conversion76 : DataTypeConversion  OutDataTypeStr=single  RndMeth=Nearest  SampleTime=1e-08  SaturateOnIntegerOverflow=off
  Data Type Conversion76_pd1 : Delay  DelayLength=6
  Out1 : Outport
  wires:
  In1/1 -> Data Type Conversion76/1
  Data Type Conversion76/1 -> Data Type Conversion76_pd1/1
  Data Type Conversion76_pd1/1 -> Out1/1

== system gm_parallel_8_prediction_and_cost_function/Prediction_and_cost_function1/Data Type Conversion77 ==
  In1 : Inport
  Data Type Conversion77 : DataTypeConversion  OutDataTypeStr=single  RndMeth=Nearest  SampleTime=1e-08  SaturateOnIntegerOverflow=off
  Data Type Conversion77_pd1 : Delay  DelayLength=6
  Out1 : Outport
  wires:
  In1/1 -> Data Type Conversion77/1
  Data Type Conversion77/1 -> Data Type Conversion77_pd1/1
  Data Type Conversion77_pd1/1 -> Out1/1

== system gm_parallel_8_prediction_and_cost_function/Prediction_and_cost_function1/Data Type Conversion8 ==
  In1 : Inport
  Data Type Conversion8 : DataTypeConversion  OutDataTypeStr=single  RndMeth=Nearest  SampleTime=1e-08  SaturateOnIntegerOverflow=off
  Data Type Conversion8_pd1 : Delay  DelayLength=6
  Out1 : Outport
  wires:
  In1/1 -> Data Type Conversion8/1
  Data Type Conversion8/1 -> Data Type Conversion8_pd1/1
  Data Type Conversion8_pd1/1 -> Out1/1

== system gm_parallel_8_prediction_and_cost_function/Prediction_and_cost_function1/Data Type Conversion9 ==
  In1 : Inport
  Data Type Conversion9 : DataTypeConversion  OutDataTypeStr=single  RndMeth=Nearest  SampleTime=1e-08  SaturateOnIntegerOverflow=off
  Data Type Conversion9_pd1 : Delay  DelayLength=6
  Out1 : Outport
  wires:
  In1/1 -> Data Type Conversion9/1
  Data Type Conversion9/1 -> Data Type Conversion9_pd1/1
  Data Type Conversion9_pd1/1 -> Out1/1

== system gm_parallel_8_prediction_and_cost_function/Prediction_and_cost_function1/Detect Rise Positive ==
  note: Edge
  note: U(k)
  U : Inport  OutDataTypeStr=boolean  SampleTime=1e-08
  Delay Input1 : UnitDelay  Description=Store in Global RAM  DisableCoverage=on  InitialCondition=vinit  SampleTime=-1  HasFrameUpgradeWarning=on
  FixPt Relational Operator : RelationalOperator  Operator=>  OutDataTypeStr=boolean  ZeroCross=off  InputSameDT=off
  Positive : Subsystem  mask(Compare To Zero){relop=>, OutDataTypeStr=boolean, ZeroCross=off}
      mask prompts: relop "Simulink:masks:Operator_MP"; OutDataTypeStr "Simulink:masks:OutputDataType_MP"; ZeroCross "Simulink:masks:EnableZerocrossingDetection_MP"
      mask help: Simulink:masks:CompareToZero_MD
      mask init:
      | OutDataTypeStr = 'boolean';
      | ZeroCross = 'off';
      | blkName = 'parallel_8_prediction_and_cost_function/Prediction_and_cost_function1/Detect Rise\nPositive/Positive';
      | relop = '>';
      | setValue = 'boolean';
      mask TypeOptions relop: == | ~= | < | <= | >= | >
      mask TypeOptions OutDataTypeStr: Simulink:masks:uint8 | Simulink:masks:boolean
      mask Callback ZeroCross: sl('zeroCrossEnable', gcbh);
      mask Display: disp([relop,' 0'])
  Y : Outport  SampleTime=1e-08
  wires:
  Delay Input1/1 -> FixPt Relational Operator/2
  FixPt Relational Operator/1 -> Y/1
  Positive/1(y) -> FixPt Relational Operator/1, Delay Input1/1
  U/1 -> Positive/1(u)

== system gm_parallel_8_prediction_and_cost_function/Prediction_and_cost_function1/Detect Rise Positive1 ==
  note: Edge
  note: U(k)
  U : Inport  OutDataTypeStr=boolean  SampleTime=1e-08
  Delay Input1 : UnitDelay  Description=Store in Global RAM  DisableCoverage=on  InitialCondition=vinit  SampleTime=-1  HasFrameUpgradeWarning=on
  FixPt Relational Operator : RelationalOperator  Operator=>  OutDataTypeStr=boolean  ZeroCross=off  InputSameDT=off
  Positive : Subsystem  mask(Compare To Zero){relop=>, OutDataTypeStr=boolean, ZeroCross=off}
      mask prompts: relop "Simulink:masks:Operator_MP"; OutDataTypeStr "Simulink:masks:OutputDataType_MP"; ZeroCross "Simulink:masks:EnableZerocrossingDetection_MP"
      mask help: Simulink:masks:CompareToZero_MD
      mask init:
      | OutDataTypeStr = 'boolean';
      | ZeroCross = 'off';
      | blkName = 'parallel_8_prediction_and_cost_function/Prediction_and_cost_function1/Detect Rise\nPositive1/Positive';
      | relop = '>';
      | setValue = 'boolean';
      mask TypeOptions relop: == | ~= | < | <= | >= | >
      mask TypeOptions OutDataTypeStr: Simulink:masks:uint8 | Simulink:masks:boolean
      mask Callback ZeroCross: sl('zeroCrossEnable', gcbh);
      mask Display: disp([relop,' 0'])
  Y : Outport  SampleTime=1e-08
  wires:
  Delay Input1/1 -> FixPt Relational Operator/2
  FixPt Relational Operator/1 -> Y/1
  Positive/1(y) -> FixPt Relational Operator/1, Delay Input1/1
  U/1 -> Positive/1(u)

== system gm_parallel_8_prediction_and_cost_function/Prediction_and_cost_function1/Detect Rise Positive2 ==
  note: Edge
  note: U(k)
  U : Inport  OutDataTypeStr=boolean  SampleTime=1e-08
  Delay Input1 : UnitDelay  Description=Store in Global RAM  DisableCoverage=on  InitialCondition=vinit  SampleTime=-1  HasFrameUpgradeWarning=on
  FixPt Relational Operator : RelationalOperator  Operator=>  OutDataTypeStr=boolean  ZeroCross=off  InputSameDT=off
  Positive : Subsystem  mask(Compare To Zero){relop=>, OutDataTypeStr=boolean, ZeroCross=off}
      mask prompts: relop "Simulink:masks:Operator_MP"; OutDataTypeStr "Simulink:masks:OutputDataType_MP"; ZeroCross "Simulink:masks:EnableZerocrossingDetection_MP"
      mask help: Simulink:masks:CompareToZero_MD
      mask init:
      | OutDataTypeStr = 'boolean';
      | ZeroCross = 'off';
      | blkName = 'parallel_8_prediction_and_cost_function/Prediction_and_cost_function1/Detect Rise\nPositive2/Positive';
      | relop = '>';
      | setValue = 'boolean';
      mask TypeOptions relop: == | ~= | < | <= | >= | >
      mask TypeOptions OutDataTypeStr: Simulink:masks:uint8 | Simulink:masks:boolean
      mask Callback ZeroCross: sl('zeroCrossEnable', gcbh);
      mask Display: disp([relop,' 0'])
  Y : Outport  SampleTime=1e-08
  wires:
  Delay Input1/1 -> FixPt Relational Operator/2
  FixPt Relational Operator/1 -> Y/1
  Positive/1(y) -> FixPt Relational Operator/1, Delay Input1/1
  U/1 -> Positive/1(u)

== system gm_parallel_8_prediction_and_cost_function/Prediction_and_cost_function1/Product ==
  In1 : Inport
  In2 : Inport  Port=2
  Product : Product  Inputs=**  OutDataTypeStr=single  SampleTime=1e-08
  Product_pd1 : Delay  DelayLength=6
  Out1 : Outport
  wires:
  In1/1 -> Product/1
  In2/1 -> Product/2
  Product/1 -> Product_pd1/1
  Product_pd1/1 -> Out1/1
